simulink model "gdnn_lm_rtrl"  (R2018a)
settings: Solver=ode5  StartTime=0.0  StopTime=train_length  FixedStep=T_sim  RelTol=1e-3  EnableMultiTasking=on
values from neighbouring files (symbols this model uses):
  bb = zeros(1,numoflayers)    [ini_gdnn.m]
  bs = zeros(1,numoflayers)    [ini_gdnn.m]
  D_max = max(max(max(max(idel))),max(max(max(ldel))))    [ini_gdnn.m]
  DI_vec = [DI_vec DI(i,:)]    [ini_gdnn.m]
  DIB_vec = [DIB_vec DIB(i,:)]    [ini_gdnn.m]
  dimax = max(dimax)    [ini_gdnn.m]
  DIS_vec = [DIS_vec DIS(i,:)]    [ini_gdnn.m]
  DL_vec = [DL_vec DL(i,:)]    [ini_gdnn.m]
  DLB_vec = [DLB_vec DLB(i,:)]    [ini_gdnn.m]
  dlmax = max(dlmax)    [ini_gdnn.m]
  DLS_vec = [DLS_vec DLS(i,:)]    [ini_gdnn.m]
  E_LW_U = zeros(1,numoflayers^2)    [ini_gdnn.m]
  gamma = 1    [ini_gdnn.m]
  I = zeros(1,numoflayers*numofinputs)    [ini_gdnn.m]
  idelb_vec = 0    [ini_gdnn.m]
  idels_vec = 0    [ini_gdnn.m]
  Lb = zeros(1,numoflayers^2)    [ini_gdnn.m]
  ldelb_vec = 0    [ini_gdnn.m]
  ldels_vec = 0    [ini_gdnn.m]
  Lf = zeros(1,numoflayers^2)    [ini_gdnn.m]
  net_params = [Q, mue, theta, T, L, D_max, numoflayers, numofinputs, max(S), sum(R), S_out, S_target, print_weights, min_weights, prune_interval, train_length, prune_maxerr_OBS, prune_maxerr_exact]    [ini_gdnn.m]
  omega_d = 1    [ini_gdnn.m]
  Q = 50    [ini_gdnn.m]
  switch_input = 1    [ini_gdnn.m]
  switch_input_wave = 1    [ini_gdnn.m]
  sys_switch = 1    [ini_gdnn.m]
  T = 0.01    [ini_gdnn.m]
  train_length = 15    [Auswertung.m]    (also in ini_gdnn.m = 5000)
  U = U_target    [ini_gdnn.m]
  U_out = zeros(1,numoflayers)    [ini_gdnn.m]
  U_target = zeros(1,numoflayers)    [ini_gdnn.m]
  W_alpha_ini = ones(1,L)    [ini_gdnn.m]
  W_ini = rand(1,L) - 0.5    [ini_gdnn.m]
  X = zeros(1,numoflayers)    [ini_gdnn.m]
undefined symbols (not defined in the file or in its folder): idel_vec, ldel_vec, R, S
libraries: simulink x3
CloseFcn:
  | rtwprivate ssgencode ModelCloseRequest gdnn_lm_rtrl
settings Model: Creator=endisch  LastModifiedBy=Maxi
settings DataIOCC: LimitDataPoints=on  SaveFormat=Array  SignalLoggingSaveFormat=ModelDataLogs
settings OptimizationCC: InitFltsAndDblsToZero=on  LifeSpan=inf
settings DebuggingCC: SaveWithParameterizedLinksMsg=none  UnderspecifiedInitializationDetection=Classic  MergeDetectMultiDrivingBlocksExec=none  SignalResolutionControl=TryResolveAllWithWarning  SolverPrmCheckMsg=warning  MultiTaskDSMMsg=warning  MultiTaskCondExecSysMsg=none  FcnCallInpInsideContextMsg=warning  AllowSymbolicDim=off  StateNameClashWarn=warning  SFUnexpectedBacktrackingDiag=warning  SFNoUnconditionalDefaultTransitionDiag=warning  SFExecutionAtInitializationDiag=none
settings HardwareCC: ProdBitPerPointer=32  ProdBitPerSizeT=32  ProdBitPerPtrDiffT=32  ProdLargestAtomicFloat=None  ProdIntDivRoundTo=Undefined  ProdEndianess=Unspecified  ProdWordSize=32  ProdHWDeviceType=32-bit Generic
settings ModelReferenceCC: PropagateSignalLabelsOutOfModel=off
settings CodeAppCC: StateflowObjectComments=on
settings GRTTargetCC: TargetFcnLib=ansi_tfl_tmw.mat  TargetLangStandard=C89/C90 (ANSI)  GeneratePreprocessorConditionals=Disable all  CombineOutputUpdateFcns=off  GRTInterface=on
settings ConfigComp: CovMetricSettings=dw  CovHtmlReporting=on  CovSaveCumulativeToWorkspaceVar=on  CovSaveSingleToWorkspaceVar=on  CovExternalEMLEnable=off

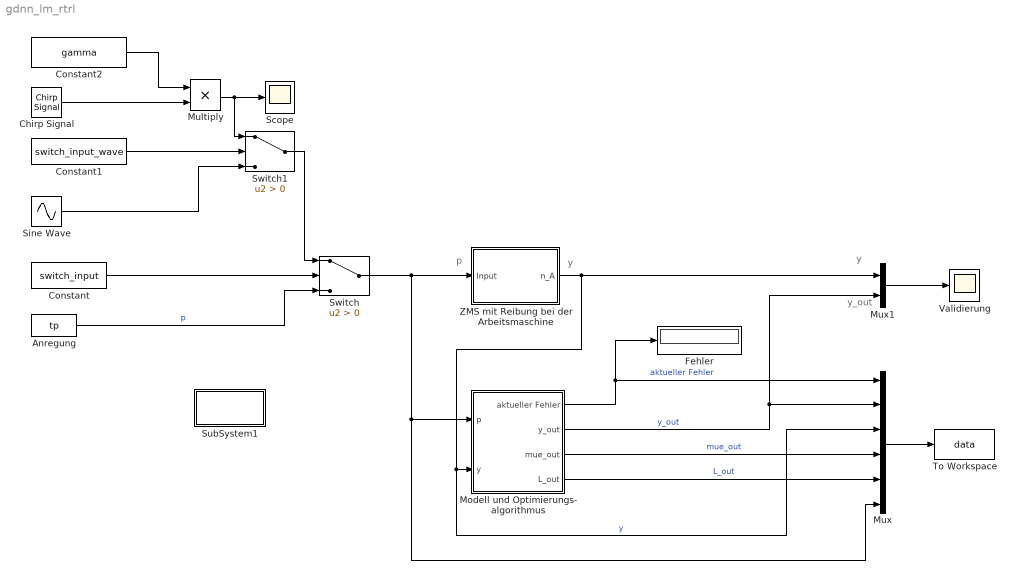
== system gdnn_lm_rtrl ==
  note: y_out
  note: y
  note: y
  note: p
  Anregung : FromWorkspace  VariableName=tp  SampleTime=T  Interpolate=off  OutputAfterFinalValue=Cyclic repetition
  Chirp Signal : simulink/Sources/Chirp Signal  f1=Freq_init  T=train_length  f2=Freq_max
  Constant : Constant  Value=switch_input
  Constant1 : Constant  Value=switch_input_wave
  Constant2 : Constant  Value=gamma
  Fehler : Display
      settings: Format=short_e
  Modell und Optimierungs- algorithmus : Subsystem
  Multiply : Product
  Mux : Mux  Inputs=6
  Mux1 : Mux  Inputs=2
  Scope : Scope
  Sine Wave : Sin  Amplitude=gamma  Frequency=omega_d  SampleTime=T
  SubSystem1 : Subsystem
      settings: OpenFcn=ini_gdnn
      mask Display: disp('Initialize\n(Double-Click)')
  Switch : Switch  Criteria=u2 > Threshold
  Switch1 : Switch  Criteria=u2 > Threshold
  To Workspace : ToWorkspace  VariableName=data  SaveFormat=Structure With Time  SampleTime=-1
  Validierung : Scope
  ZMS mit Reibung bei der Arbeitsmaschine : Subsystem
  wires:
  Mux/1 -> To Workspace/1
  ZMS mit Reibung bei der Arbeitsmaschine/1(n_A) -> Mux/3, Modell und Optimierungs- algorithmus/2(y), Mux1/1  "y"
  Anregung/1 -> Switch/3  "p"
  Modell und Optimierungs- algorithmus/1(aktueller Fehler) -> Fehler/1, Mux/1  "aktueller Fehler"
  Modell und Optimierungs- algorithmus/3(mue_out) -> Mux/4  "mue_out"
  Modell und Optimierungs- algorithmus/4(L_out) -> Mux/5  "L_out"
  Mux1/1 -> Validierung/1
  Modell und Optimierungs- algorithmus/2(y_out) -> Mux/2, Mux1/2  "y_out"
  Switch/1 -> Mux/6, Modell und Optimierungs- algorithmus/1(p), ZMS mit Reibung bei der Arbeitsmaschine/1(Input)
  Constant/1 -> Switch/2
  Constant1/1 -> Switch1/2
  Sine Wave/1 -> Switch1/3
  Switch1/1 -> Switch/1
  Chirp Signal/1 -> Multiply/2
  Multiply/1 -> Switch1/1, Scope/1
  Constant2/1 -> Multiply/1

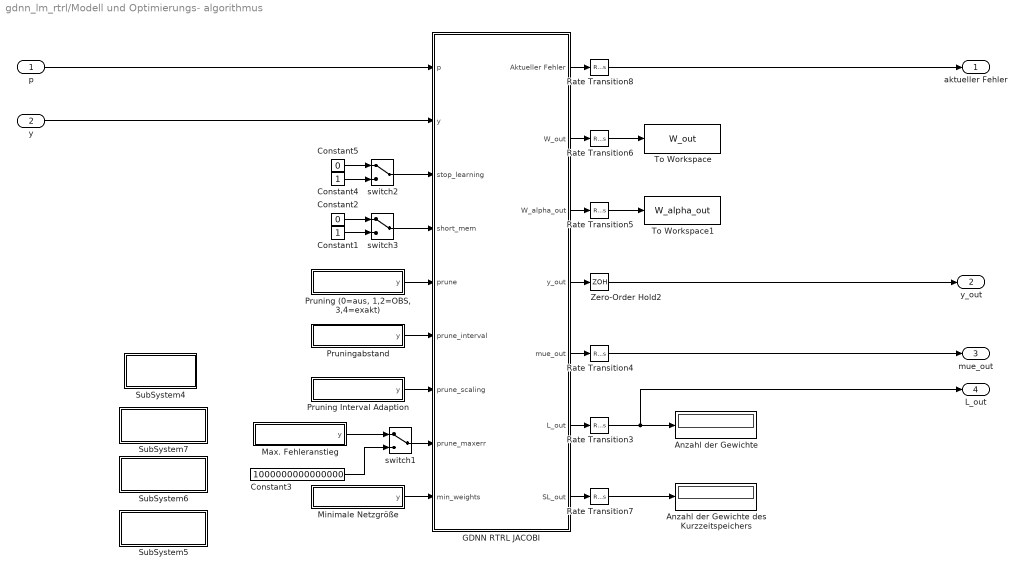
== system gdnn_lm_rtrl/Modell und Optimierungs- algorithmus ==
  p : Inport
  y : Inport  Port=2
  Anzahl der Gewichte : Display
  Anzahl der Gewichte des Kurzzeitspeichers : Display
  Constant1 : Constant
  Constant2 : Constant  Value=0
  Constant3 : Constant  Value=1000000000000000
  Constant4 : Constant
  Constant5 : Constant  Value=0
  GDNN RTRL JACOBI : Subsystem  TreatAsAtomicUnit=on  SystemSampleTime=T
  Max. Fehleranstieg : Subsystem  TreatAsAtomicUnit=on  SystemSampleTime=T  mask(Max. Error After Pruning-Step){number=10}
      mask prompts: number "Max. zulässig ist alter Fehler mal:"
      mask help: 0: Slider inaktiv, Wert wird aus der Ini-Datei (ini_gdnn.m) genommen
      mask Display: disp(sprintf('Fehleranstieg: %.1f',number));
  Minimale Netzgröße : Subsystem  TreatAsAtomicUnit=on  SystemSampleTime=T  mask(Minimum Number of Weights){number=1}
      mask prompts: number "Minimale Anzahl an Gewichte:"
      mask help: 0: Slider inaktiv, Wert wird aus der Ini-Datei (ini_gdnn.m) genommen
      mask Display: disp(sprintf('Gewichte: %i',number));
  "Pruning (0=aus, 1,2=OBS, 3,4=exakt)" : Subsystem  TreatAsAtomicUnit=on  SystemSampleTime=T  mask(Pruning Algorithms){number=0}
      mask prompts: number "Pruningverfahren:"
      mask help:
      | 0: aus
      | 1: OBS
      | 2: OBS, Berücksichtigung der Verzögerungsordnung
      | 3: exaktes Pruning
      | 4: exaktes Pruning, Berücksichtigung der Verzögerungsordnung
      mask TypeOptions number: 0 | 1 | 2 | 3 | 4
      mask Display: disp(sprintf('pruning %i',number-1));
  Pruning Interval Adaption : Subsystem  TreatAsAtomicUnit=on  SystemSampleTime=T  mask(Pruning Interval adaption){number=1}
      mask prompts: number "Skalierungsfaktor"
      mask help: 1.0: Pruning Interval wird nicht angepasst, Pruning Interval ist konstant
      mask Display: disp(sprintf('Scaling: %.1f',number));
  Pruningabstand : Subsystem  TreatAsAtomicUnit=on  SystemSampleTime=T  mask(Pruning Interval){number=100}
      mask prompts: number "Intervall (Abstand zweier Pruningschritte):"
      mask help: 0: Slider inaktiv, Wert wird aus der Ini-Datei (ini_gdnn.m) genommen
      mask Display: disp(sprintf('Intervall: %i',number));
  Rate Transition{3..8} (6 alike) : RateTransition  OutPortSampleTime=T
  SubSystem4 : Subsystem
      settings: OpenFcn=clc
      mask Display: disp('Clear screen\n(Double-Click)')
  SubSystem5 : Subsystem
      settings: OpenFcn=|
      | net_params2 = net_params;
      | Q2=Q;
      | D_max2=D_max;
      | 
      | 
      | R2 = R;
      | S2 = S;
      | U2 = U;
      | X2 = X;
      | I2 = I;
      | Lf2 = Lf;
      | Lb2 = Lb;
      | E_LW_U2 = E_LW_U;
      | DI_vec2 = DI_vec;
      | DL_vec2 = DL_vec;
      | dimax2 = dimax;
      | dlmax2 = dlmax;
      | U_out2 = U_out;
      | U_target2 = U_target;
      | W_ini2 = W_out;
      | W_alpha_ini2 = W_alpha_out;
      | idel_vec2 = idel_vec;
      | ldel_vec2 = ldel_vec;
      | 
      | DIS_vec2=DIS_vec;
      | 
      | DLS_vec2=DLS_vec;
      | 
      | idels_vec2=idels_vec;
      | 
      | ldels_vec2=ldels_vec;
      | 
      | bs2=bs;
      | 
      | DIB_vec2=DIB_vec;
      | 
      | DLB_vec2=DLB_vec;
      | 
      | idelb_vec2=idelb_vec;
      | 
      | ldelb_vec2=ldelb_vec;
      | 
      | bb2= bb;
      | 
      | if exist('params.mat','file') ~= 0
      | !del params.mat
      | end
      | save params net_params2 Q2 D_max2 R2 S2 U2 X2 I2 Lf2 Lb2 E_LW_U2 DI_vec2 DL_vec2 dimax2 dlmax2 U_out2 U_target2 W_ini2 W_alpha_ini2 idel_vec2 ldel_vec2 DIS_vec2 DLS_vec2 idels_vec2 ldels_vec2 bs2 DIB_vec2 DLB_vec2 idelb_vec2 ldelb_vec2 bb2 ;
      | 
      | !copy params.mat ..\11.04.07Gesamtmodell\params.mat
      mask Display: disp('Create params.mat\n(Double-Click)')
  SubSystem6 : Subsystem
      settings: OpenFcn=save W W_out W_alpha_out;
      mask Display: disp('Save weights\n(Double-Click)')
  SubSystem7 : Subsystem
      settings: OpenFcn=|
      | load W;
      | W_ini=W_out;
      | W_alpha_ini=W_alpha_out;
      mask Display: disp('Load old weights\n(Double-Click)')
  To Workspace : ToWorkspace  VariableName=W_out  SampleTime=T
      settings: MaxDataPoints=1
  To Workspace1 : ToWorkspace  VariableName=W_alpha_out  SampleTime=T
      settings: MaxDataPoints=1
  Zero-Order Hold2 : ZeroOrderHold  SampleTime=T
  switch1 : ManualSwitch
  switch2 : ManualSwitch
  switch3 : ManualSwitch
  aktueller Fehler : Outport
  y_out : Outport  Port=2
  mue_out : Outport  Port=3
  L_out : Outport  Port=4
  wires:
  p/1 -> GDNN RTRL JACOBI/1(p)
  y/1 -> GDNN RTRL JACOBI/2(y)
  Constant4/1 -> switch2/2
  Rate Transition8/1 -> aktueller Fehler/1
  switch3/1 -> GDNN RTRL JACOBI/4(short_mem)
  GDNN RTRL JACOBI/4(y_out) -> Zero-Order Hold2/1
  "Pruning (0=aus, 1,2=OBS, 3,4=exakt)"/1(y) -> GDNN RTRL JACOBI/5(prune)
  Minimale Netzgröße/1(y) -> GDNN RTRL JACOBI/9(min_weights)
  Rate Transition7/1 -> Anzahl der Gewichte des Kurzzeitspeichers/1
  GDNN RTRL JACOBI/1(Aktueller Fehler) -> Rate Transition8/1
  GDNN RTRL JACOBI/6(L_out) -> Rate Transition3/1
  Pruning Interval Adaption/1(y) -> GDNN RTRL JACOBI/7("prune_scaling ")
  GDNN RTRL JACOBI/5(mue_out) -> Rate Transition4/1
  Constant2/1 -> switch3/1
  Rate Transition3/1 -> L_out/1, Anzahl der Gewichte/1
  Rate Transition5/1 -> To Workspace1/1
  Constant3/1 -> switch1/2
  GDNN RTRL JACOBI/3(W_alpha_out) -> Rate Transition5/1
  Rate Transition4/1 -> mue_out/1
  Constant5/1 -> switch2/1
  Constant1/1 -> switch3/2
  Zero-Order Hold2/1 -> y_out/1
  switch1/1 -> GDNN RTRL JACOBI/8(prune_maxerr)
  Rate Transition6/1 -> To Workspace/1
  Pruningabstand/1(y) -> GDNN RTRL JACOBI/6("prune_interval ")
  GDNN RTRL JACOBI/2(W_out) -> Rate Transition6/1
  GDNN RTRL JACOBI/7(SL_out) -> Rate Transition7/1
  Max. Fehleranstieg/1(y) -> switch1/1
  switch2/1 -> GDNN RTRL JACOBI/3(stop_learning)

== system gdnn_lm_rtrl/SubSystem1 ==

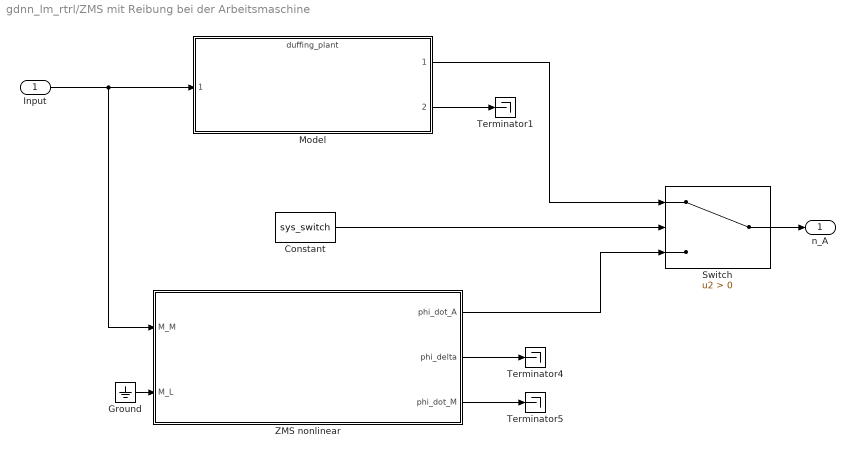
== system gdnn_lm_rtrl/ZMS mit Reibung bei der Arbeitsmaschine ==
  Input : Inport
  Constant : Constant  Value=sys_switch
  Ground : Ground
  Model : ModelReference  ModelNameDialog=duffing_plant.slx  SimulationMode=Normal  ModelReferenceVersion=1.34
  Switch : Switch  Criteria=u2 > Threshold
  Terminator1 : Terminator
  Terminator4 : Terminator
  Terminator5 : Terminator
  ZMS nonlinear : Subsystem  AncestorBlock=mytoolbox/ZMS/Linear/ZMS  mask(ZMS (linear)){c=410, d=0.5, Theta_M=0.333, Theta_A=0.166, ue=1, mue_1=0.5, mue_2=25, mue_3=1, mue_4=0.2, mue_5=1, mue_6=0.03}
      mask prompts: c "Stiffness of Shaft c"; d "Damping of Shaft d"; Theta_M "Inertia of Motor Theta_M"; Theta_A "Inertia of Load Theta_A"; ue "Transmission Ratio ue"
      mask help:
      | This blocks includes a model of a linear flexible two-mass system (ZMS)
      | without friction or backlash behaviour. Used Parameters:
      | c			"Stiffness"
      | d			"Damping"
      | Theta_M		"Inertia of Motor"
      | Theta_A		"Inertia of Load"
      | ue			"Transmission Ratio"
      mask Display:
      | port_label('input',1,sprintf('Motor Torque M_M'));
      | port_label('input',2,sprintf('Load Torque M_L'));
      | 
      | port_label('output',1,sprintf('Load speed Omega_A'));
      | port_label('output',2,sprintf('Angle of Twist Delta_phi'));
      | port_label('output',3,sprintf('Motor speed Omega_M'));
      | 
      | disp(sprintf('ZMS nonlinear'))
  n_A : Outport
  wires:
  ZMS nonlinear/2(phi_delta) -> Terminator4/1
  ZMS nonlinear/3(phi_dot_M) -> Terminator5/1
  Ground/1 -> ZMS nonlinear/2(M_L)
  Input/1 -> ZMS nonlinear/1(M_M), Model/1
  Model/2 -> Terminator1/1
  Switch/1 -> n_A/1
  Constant/1 -> Switch/2
  ZMS nonlinear/1(phi_dot_A) -> Switch/3
  Model/1 -> Switch/1

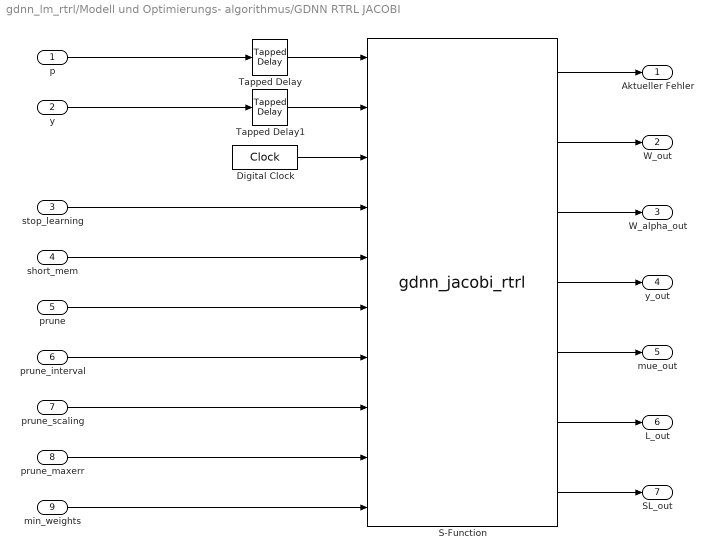
== system gdnn_lm_rtrl/Modell und Optimierungs- algorithmus/GDNN RTRL JACOBI ==
  p : Inport
  y : Inport  Port=2
  stop_learning : Inport  Port=3
  short_mem : Inport  Port=4
  prune : Inport  Port=5
  "prune_interval " : Inport  Port=6
  "prune_scaling " : Inport  Port=7
  prune_maxerr : Inport  Port=8
  min_weights : Inport  Port=9
  Digital Clock : DigitalClock  SampleTime=T
  S-Function : S-Function  FunctionName=gdnn_jacobi_rtrl  Parameters=net_params,R,S,U,X,I,Lf,Lb,E_LW_U,DI_vec,DL_vec,dimax,dlmax,U_out,U_target,W_ini,W_alpha_ini,idel_vec,ldel_vec,DIS_vec,DLS_vec,idels_vec,ldels_vec,bs,DIB_vec,DLB_vec,idelb_vec,ldelb_vec,bb  SFunctionModules=forward_step.c get_jacobi_rtrl.c w_conv.c shift.c transfer.c m_inv.c pruning1_4.c mem_alloc.c mem_free.c  SFunctionDeploymentMode=off  EnableBusSupport=off
  Tapped Delay : simulink/Discrete/Tapped Delay  vinit=0.0  samptime=-1  NumDelays=Q+D_max-1  DelayOrder=Oldest  includeCurrent=on
  Tapped Delay1 : simulink/Discrete/Tapped Delay  vinit=0.0  samptime=-1  NumDelays=Q-1  DelayOrder=Oldest  includeCurrent=on
  Aktueller Fehler : Outport
  W_out : Outport  Port=2
  W_alpha_out : Outport  Port=3
  y_out : Outport  Port=4
  mue_out : Outport  Port=5
  L_out : Outport  Port=6
  SL_out : Outport  Port=7
  wires:
  Digital Clock/1 -> S-Function/3
  S-Function/1 -> Aktueller Fehler/1
  S-Function/2 -> W_out/1
  S-Function/3 -> W_alpha_out/1
  S-Function/4 -> y_out/1
  S-Function/5 -> mue_out/1
  S-Function/6 -> L_out/1
  S-Function/7 -> SL_out/1
  stop_learning/1 -> S-Function/4
  short_mem/1 -> S-Function/5
  prune/1 -> S-Function/6
  "prune_interval "/1 -> S-Function/7
  "prune_scaling "/1 -> S-Function/8
  prune_maxerr/1 -> S-Function/9
  min_weights/1 -> S-Function/10
  y/1 -> Tapped Delay1/1
  Tapped Delay/1 -> S-Function/1
  Tapped Delay1/1 -> S-Function/2
  p/1 -> Tapped Delay/1

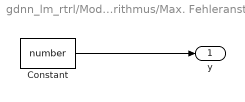
== system gdnn_lm_rtrl/Modell und Optimierungs- algorithmus/Max. Fehleranstieg ==
  Constant : Constant  Value=number
  y : Outport
  wires:
  Constant/1 -> y/1

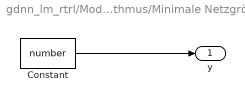
== system gdnn_lm_rtrl/Modell und Optimierungs- algorithmus/Minimale Netzgröße ==
  Constant : Constant  Value=number
  y : Outport
  wires:
  Constant/1 -> y/1

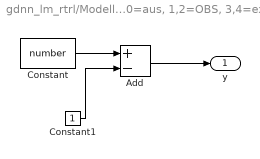
== system gdnn_lm_rtrl/Modell und Optimierungs- algorithmus/Pruning (0=aus, 1,2=OBS, 3,4=exakt) ==
  Add : Sum  Inputs=+-
  Constant : Constant  Value=number
  Constant1 : Constant
  y : Outport
  wires:
  Constant/1 -> Add/1
  Add/1 -> y/1
  Constant1/1 -> Add/2

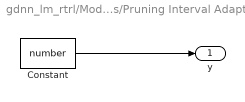
== system gdnn_lm_rtrl/Modell und Optimierungs- algorithmus/Pruning Interval Adaption ==
  Constant : Constant  Value=number
  y : Outport
  wires:
  Constant/1 -> y/1

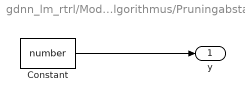
== system gdnn_lm_rtrl/Modell und Optimierungs- algorithmus/Pruningabstand ==
  Constant : Constant  Value=number
  y : Outport
  wires:
  Constant/1 -> y/1

== system gdnn_lm_rtrl/Modell und Optimierungs- algorithmus/SubSystem4 ==

== system gdnn_lm_rtrl/Modell und Optimierungs- algorithmus/SubSystem5 ==

== system gdnn_lm_rtrl/Modell und Optimierungs- algorithmus/SubSystem6 ==

== system gdnn_lm_rtrl/Modell und Optimierungs- algorithmus/SubSystem7 ==

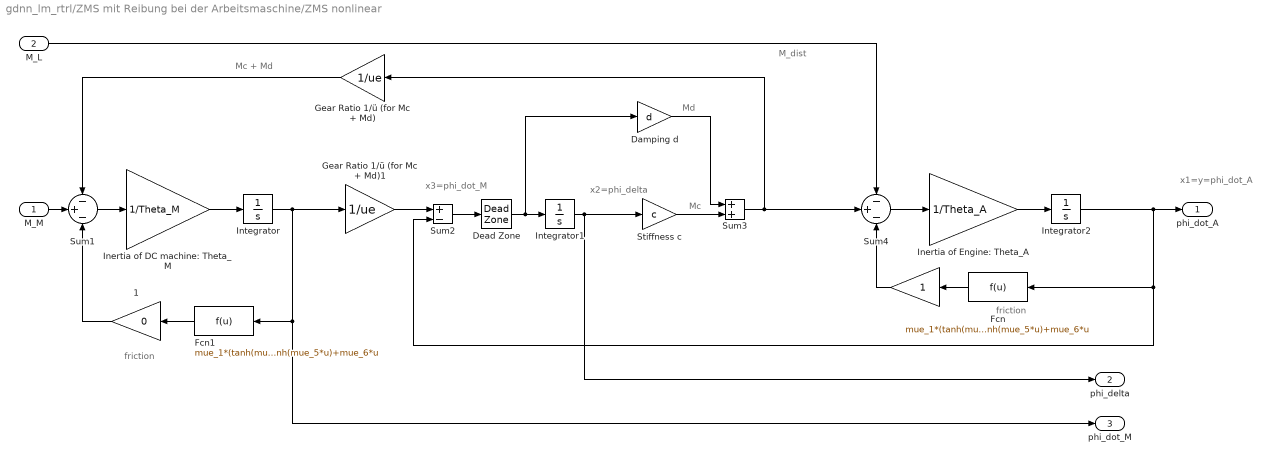
== system gdnn_lm_rtrl/ZMS mit Reibung bei der Arbeitsmaschine/ZMS nonlinear ==
  note: x3=phi_dot_M
  note: x2=phi_delta
  note: Mc + Md
  note: Md
  note: Mc
  note: M_dist
  note: x1=y=phi_dot_A
  note: friction
  note: friction
  M_M : Inport
  M_L : Inport  Port=2
  " " : Gain  SaturateOnIntegerOverflow=on  OutDataTypeStr=Inherit: Same as input  ParamDataTypeStr=Inherit: Same as input
  " 1" : Gain  Gain=0  SaturateOnIntegerOverflow=on  OutDataTypeStr=Inherit: Same as input  ParamDataTypeStr=Inherit: Same as input
  Damping d : Gain  Gain=d  SaturateOnIntegerOverflow=on  OutDataTypeStr=Inherit: Same as input  ParamDataTypeStr=Inherit: Same as input
  Dead Zone : DeadZone  LowerValue=-0  UpperValue=0  SaturateOnIntegerOverflow=on
  Fcn : Fcn  Expr=mue_1*(tanh(mue_2*u)-tanh(mue_3*u))+mue_4*tanh(mue_5*u)+mue_6*u
  Fcn1 : Fcn  Expr=mue_1*(tanh(mue_2*u)-tanh(mue_3*u))+mue_4*tanh(mue_5*u)+mue_6*u
  Gear Ratio 1/ü (for Mc + Md) : Gain  Gain=1/ue  SaturateOnIntegerOverflow=on  OutDataTypeStr=Inherit: Same as input  ParamDataTypeStr=Inherit: Same as input
  Gear Ratio 1/ü (for Mc + Md)1 : Gain  Gain=1/ue  SaturateOnIntegerOverflow=on  OutDataTypeStr=Inherit: Same as input  ParamDataTypeStr=Inherit: Same as input
  Inertia of DC machine: Theta_M : Gain  Gain=1/Theta_M  SaturateOnIntegerOverflow=on  OutDataTypeStr=Inherit: Same as input  ParamDataTypeStr=Inherit: Same as input
  Inertia of Engine: Theta_A : Gain  Gain=1/Theta_A  SaturateOnIntegerOverflow=on  OutDataTypeStr=Inherit: Same as input  ParamDataTypeStr=Inherit: Same as input
  Integrator : Integrator
  Integrator1 : Integrator
  Integrator2 : Integrator
  Stiffness c : Gain  Gain=c  SaturateOnIntegerOverflow=on  OutDataTypeStr=Inherit: Same as input  ParamDataTypeStr=Inherit: Same as input
  Sum1 : Sum  Inputs=-+-  SaturateOnIntegerOverflow=on
  Sum2 : Sum  Inputs=+-  SaturateOnIntegerOverflow=on
  Sum3 : Sum  SaturateOnIntegerOverflow=on
  Sum4 : Sum  Inputs=-+-  SaturateOnIntegerOverflow=on
  phi_dot_A : Outport
  phi_delta : Outport  Port=2
  phi_dot_M : Outport  Port=3
  wires:
  Sum1/1 -> Inertia of DC machine: Theta_M/1
  Inertia of DC machine: Theta_M/1 -> Integrator/1
  Integrator2/1 -> phi_dot_A/1, Sum2/2, Fcn/1
  Integrator/1 -> Gear Ratio 1/ü (for Mc + Md)1/1, phi_dot_M/1, Fcn1/1
  Sum2/1 -> Dead Zone/1
  Integrator1/1 -> phi_delta/1, Stiffness c/1
  Stiffness c/1 -> Sum3/2
  Damping d/1 -> Sum3/1
  Sum3/1 -> Sum4/2, Gear Ratio 1/ü (for Mc + Md)/1
  M_L/1 -> Sum4/1
  Sum4/1 -> Inertia of Engine: Theta_A/1
  Inertia of Engine: Theta_A/1 -> Integrator2/1
  M_M/1 -> Sum1/2
  Gear Ratio 1/ü (for Mc + Md)/1 -> Sum1/1
  Gear Ratio 1/ü (for Mc + Md)1/1 -> Sum2/1
  Fcn/1 -> " "/1
  " "/1 -> Sum4/3
  Fcn1/1 -> " 1"/1
  " 1"/1 -> Sum1/3
  Dead Zone/1 -> Integrator1/1, Damping d/1
